simulink model "eVTOL_System"  (R2024b)
settings: Solver=FixedStepAuto  StartTime=0.0  StopTime=inf  RelTol=1e-3
undefined symbols (not defined in the file): airspeed, Battery, BCE12, BCE_Set_init, BMS_Controller_State, C, Cell10_P, Cell11_P, Cell12_P, Cell13_P, Cell14_P, Cell15_P, Cell16_P, Cell17_P, Cell18_P, Cell19_P, Cell1_N, Cell1_P, Cell20_P, Cell21_P, Cell22_P, Cell23_P, Cell24_P, Cell2_P, Cell3_P, Cell4_P, Cell5_P, Cell6_P, Cell7_P, Cell8_P, Cell9_P, Charging_State, CityMission, control, controlParams, ControlSampleTime, CriticalTiltAngle, currentFactor, CV_Gain, ddx, ddy, ddz, Device_01, Device_02, DiscIntNeverNeededParam, dx, dy, dz, Earth, env, F, F28379D_ADC_MaxCount, F28379D_ADC_Vmax, FixedWingMission, flightState, Foc_Ki_IxTcpu, Foc_Ki_S, Foc_Kp_I, Foc_Kp_S, fractalcoef ... (+68)
libraries: fl_lib x1115, nesl_utility x617, slrealtimeethercatlib x217, simulink x130, canmsglib x101, speedgoatlib_IO611_obsolete x91, slpidlib x49, mcbcontrolslib x44, slrealtimeutilitieslib x35, speedgoatlib_hdlCoder_IO3xx x31, dspstat3 x24, mcbpositiondecoderlib x12
(part 4 of 31)

== system eVTOL_System/User Interface/Motor Drive User Interface ==
  note: Fault Present
  note: Hardware-in-the-Loop
      | Motor & Inverter
      | Real-Time Simulation
  note: Motor Currents [A]
  note: Model Response
  note: Kp
  note: UI Speed Command enabled
  note: Tx: Message to Controller
  note: Speed Controller PI Gain Tuning
  note: Ki
  note: Rx: Message From Controller
  note: Open A-
  note: Open C-
  note: Short AB
  note: Short B
  note: Short CA
  note: Open A+
  note: Short BC
  note: Open B-
  note: Open B+
  note: Open C+
  note: Short A
  note: Short C
  note: Inverter Faults
  note: Motor Speed [rpm]
  note: Time [s]
  note: Time [s]
  note: Time [s]
  note: Motor Speed [rpm]
  note: Encoder Count [steps]
  note: (only for switching inverter)
  note: (only short A with included bitstream)
  note: Motor Drive User Interface
  Dashboard Scope1 : DashboardScope  ShowInitialText=off  TimeSpan=0.10000000000000001  Ymin=-50  Ymax=50  ScaleAtStop=off  UpdateMode=Scroll
  Dashboard Scope2 : DashboardScope  ShowInitialText=off  TimeSpan=1  Ymin=0  Ymax=1e5  ScaleAtStop=off
  Dashboard Scope3 : DashboardScope  ShowInitialText=off  TimeSpan=10  Ymin=0  Ymax=3000  ScaleAtStop=off
  Edit : EditField  LabelPosition=Hide  ShowInitialText=on  Alignment=Center
  Edit1 : EditField  LabelPosition=Hide  ShowInitialText=on  Alignment=Center
  Faults Enabled : SliderSwitchBlock  LabelPosition=Hide
      settings: Values={{'Faults UI OFF', 'Faults UI ON'}, [0 1]}
  Gauge1 : CircularGaugeBlock  LabelPosition=Hide  ScaleMin=-1500  ScaleMax=1500
  Lamp2 : LampBlock  LabelPosition=Hide
  Lamp3 : LampBlock  LabelPosition=Hide
  Lamp4 : LampBlock  LabelPosition=Hide
  Open An : ToggleSwitchBlock  LabelPosition=Hide
      settings: Values={{'Off', 'On'}, [0 1]}
  Open Ap : ToggleSwitchBlock  LabelPosition=Hide
      settings: Values={{'Off', 'On'}, [0 1]}
  Open Bn : ToggleSwitchBlock  LabelPosition=Hide
      settings: Values={{'Off', 'On'}, [0 1]}
  Open Bp : ToggleSwitchBlock  LabelPosition=Hide
      settings: Values={{'Off', 'On'}, [0 1]}
  Open Cn : ToggleSwitchBlock  LabelPosition=Hide
      settings: Values={{'Off', 'On'}, [0 1]}
  Open Cp : ToggleSwitchBlock  LabelPosition=Hide
      settings: Values={{'Off', 'On'}, [0 1]}
  Short A : ToggleSwitchBlock  LabelPosition=Hide
      settings: Values={{'Off', 'On'}, [0 1]}
  Short AB : ToggleSwitchBlock  LabelPosition=Hide
      settings: Values={{'Off', 'On'}, [0 1]}
  Short B : ToggleSwitchBlock  LabelPosition=Hide
      settings: Values={{'Off', 'On'}, [0 1]}
  Short BC : ToggleSwitchBlock  LabelPosition=Hide
      settings: Values={{'Off', 'On'}, [0 1]}
  Short C : ToggleSwitchBlock  LabelPosition=Hide
      settings: Values={{'Off', 'On'}, [0 1]}
  Short CA : ToggleSwitchBlock  LabelPosition=Hide
      settings: Values={{'Off', 'On'}, [0 1]}
  Slider : SliderBlock  LabelPosition=Hide  ScaleMin=1e-5  ScaleMax=10  ScaleType=Log
  Slider Switch : SliderSwitchBlock  LabelPosition=Hide
      settings: Values={{'Sinus Open Loop', 'FOC Closed Loop'}, [0 1]}
  Slider Switch1 : SliderSwitchBlock  LabelPosition=Hide
      settings: Values={{'PWM OFF', 'PWM ON'}, [0 1]}
  Slider Switch2 : SliderSwitchBlock  LabelPosition=Hide
      settings: Values={{'Default Values', 'Live Tuning'}, [1 0]}
  Slider1 : SliderBlock  LabelPosition=Hide  ScaleMin=1e-5  ScaleMax=10  ScaleType=Log

== system eVTOL_System/Visualization/No Visualization ==
  UAVState : Inport
  Terminator : Terminator
  wires:
  UAVState/1 -> Terminator/1

== system eVTOL_System/Visualization/Photorealistic ==
  UAVState : Inport
  PhotorealisticHIL : Subsystem  VariantControl=Visualization==2 && str2num(get_param(['eVTOL_System/Motor Drive/SimulationVariant'], 'Value'))~=1
  PhotorealisticMIL : Subsystem  VariantControl=Visualization==2 && str2num(get_param(['eVTOL_System/Motor Drive/SimulationVariant'], 'Value'))==1

== system eVTOL_System/Visualization/Visualization ==
  UAVState : Inport
  VisualizationHIL : Subsystem  VariantControl=Visualization==1 && (str2num(get_param(['eVTOL_System/Motor Drive/SimulationVariant'], 'Value'))~=1)
  VisualizationMIL : Subsystem  VariantControl=Visualization == 1 && (str2num(get_param(['eVTOL_System/Motor Drive/SimulationVariant'], 'Value'))==1)

== system eVTOL_System/Battery System/BMS/HIL ==
  State_Request : Inport  OutDataTypeStr=Enum: SRE  PortDimensions=1
  Sensor_Values : Inport  Port=2
  Bus Creator : BusCreator  Inputs=4  OutDataTypeStr=Bus: Controller_Info  NonVirtualBus=on
      settings: InheritFromInputs=off
  Bus Creator1 : BusCreator  Inputs=3  OutDataTypeStr=Bus: Controller_Output  NonVirtualBus=on
      settings: InheritFromInputs=off
  Cell Monitoring Unit : Subsystem
  Controller_100Cells : Subsystem  VariantControl=Ns_Module == 12
  Controller_76Cells : Subsystem  Commented=on
  Rate Transition : RateTransition  OutPortSampleTime=ts_controller
  Rate Transition1 : RateTransition  InitialCondition=SRE.Standby  OutPortSampleTime=ts_controller
  Rate Transition3 : RateTransition  Commented=on  InitialCondition=SRE.Standby  OutPortSampleTime=ts_controller
  Simscape Bus : SimscapeBus
  Terminator{,1..6} (7 alike) : Terminator
  Cells : PMIOPort  Side=Left
  Cells1 : PMIOPort  Port=2  Side=Left
  Cells2 : PMIOPort  Port=3  Side=Left
  Controller_Info : Outport
  Controller_Output : Outport  Port=2  OutDataTypeStr=Bus: Controller_Output  VectorParamsAs1DForOutWhenUnconnected=off  BusOutputAsStruct=on
  wires:
  Bus Creator/1 -> Controller_Info/1  "Controller_Info"
  Bus Creator1/1 -> Controller_Output/1  "Controller_Output"
  Rate Transition/1 -> Cell Monitoring Unit/2(Sensor_Values)
  Cell Monitoring Unit/1(Sensor Values) -> Controller_100Cells/1(Sensor_Values)
  Rate Transition1/1 -> Controller_100Cells/2(State_Request)
  Controller_100Cells/1(BMS_Faults) -> Bus Creator/1
  Controller_100Cells/2(Charging_State) -> Bus Creator/2
  Controller_100Cells/3(BMS_State) -> Bus Creator/3
  Controller_100Cells/4(SOC) -> Bus Creator/4
  Controller_100Cells/5(Discharge_Current_Limit) -> Bus Creator1/1
  Controller_100Cells/6(Charge_Current_Limit) -> Bus Creator1/2
  Controller_100Cells/7(Charge_Current_Req) -> Bus Creator1/3
  State_Request/1 -> Rate Transition1/1
  Sensor_Values/1 -> Rate Transition/1
  Rate Transition3/1 -> Controller_76Cells/2(State_Request)
  Controller_76Cells/1(Faults) -> Terminator/1
  Controller_76Cells/2(Charging_State) -> Terminator1/1  "Charging_State"
  Controller_76Cells/3(BMS_Controller_State) -> Terminator2/1  "BMS_State"
  Controller_76Cells/4(SOC) -> Terminator3/1
  Controller_76Cells/5(Discharge_Current_Limit) -> Terminator4/1
  Controller_76Cells/6(Charge_Current_Limit) -> Terminator5/1
  Controller_76Cells/7(Charge_Current_Req) -> Terminator6/1
  [Bal_Cmd_Controller1] -> Cell Monitoring Unit/1(Bal_Cmd_Controller)
  Controller_100Cells/8(Bal_Cmd_76Cells) -> [Bal_Cmd_Controller1]
  connections:
  Simscape Bus/RConn1 -- Cells/RConn1
  Cells1/RConn1 -- Cell Monitoring Unit/LConn1
  Cells2/RConn1 -- Cell Monitoring Unit/LConn2

== system eVTOL_System/Battery System/BMS/MIL ==
  State_Request : Inport  OutDataTypeStr=Enum: SRE  PortDimensions=1
  Sensor_Values : Inport  Port=2  OutDataTypeStr=Bus: Sensor_Values  BusOutputAsStruct=on
  Bus Creator : BusCreator  Inputs=4  OutDataTypeStr=Bus: Controller_Info  NonVirtualBus=on
      settings: InheritFromInputs=off
  Bus Creator1 : BusCreator  Inputs=4  OutDataTypeStr=Bus: Controller_Output  NonVirtualBus=on
      settings: InheritFromInputs=off
  Cell Monitoring Unit : Subsystem
  Controller : Subsystem
  Rate Transition : RateTransition  InitialCondition=struct('Cell_Voltages',3.7*ones(Ns_Module,1),'Cell_Temperatures',298.15*ones(Ns_Module,1),'Pack_Current',0,'Pack_Voltage',3.7*Ns_Module)  OutPortSampleTime=ts_controller
  Rate Transition1 : RateTransition  InitialCondition=SRE.Standby  OutPortSampleTime=ts_controller
  Rate Transition2 : RateTransition  Commented=on  InitialCondition=struct('Cell_Voltages',3.7*ones(1,Ns_Module),'Cell_Temperatures',298.15*ones(1,Ns_Module),'Pack_Current',0,'Pack_Voltage',3.7*Ns_Module)  OutPortSampleTime=ts_controller
  Rate Transition3 : RateTransition  OutPortSampleTime=ts_system
  Rate Transition{4..7} (4 alike) : RateTransition
  Cells : PMIOPort  Side=Left
  Cells1 : PMIOPort  Port=2  Side=Left
  Cells2 : PMIOPort  Port=3  Side=Left
  Controller_Info : Outport
  Controller_Output : Outport  Port=2  OutDataTypeStr=Bus: Controller_Output  VectorParamsAs1DForOutWhenUnconnected=off  BusOutputAsStruct=on
  wires:
  Bus Creator/1 -> Controller_Info/1  "Controller_Info"
  Bus Creator1/1 -> Rate Transition3/1  "Controller_Output"
  State_Request/1 -> Rate Transition1/1
  Controller/1(Faults) -> Bus Creator/1
  Controller/2(Charging_State) -> Bus Creator/2  "Charging_State"
  Controller/3(BMS_Controller_State) -> Bus Creator/3  "BMS_State"
  Controller/4(SOC) -> Bus Creator/4
  Controller/5(Discharge_Current_Limit) -> Rate Transition7/1
  Controller/6(Charge_Current_Limit) -> Rate Transition5/1
  Controller/7(Charge_Current_Req) -> Rate Transition4/1
  Controller/8(Bal_Cmd) -> Rate Transition6/1, [Bal_Cmd_Controller]
  [Bal_Cmd_Controller] -> Cell Monitoring Unit/1(Bal_Cmd_Controller)
  Sensor_Values/1 -> Rate Transition/1
  Cell Monitoring Unit/1(Sensor Values) -> Controller/1(Sensor_Values)
  Rate Transition1/1 -> Controller/2(State_Request)
  Rate Transition/1 -> Cell Monitoring Unit/2(Sensor_Values)
  Rate Transition3/1 -> Controller_Output/1
  Rate Transition4/1 -> Bus Creator1/3
  Rate Transition6/1 -> Bus Creator1/4
  Rate Transition5/1 -> Bus Creator1/2
  Rate Transition7/1 -> Bus Creator1/1
  connections:
  Cells/RConn1 -- Cell Monitoring Unit/LConn1
  Cells1/RConn1 -- Cell Monitoring Unit/LConn2
  Cells2/RConn1 -- Cell Monitoring Unit/LConn3

== system eVTOL_System/Battery System/Battery/Battery Pack ==
  Ambient_Temperature : Inport
  100-Cell : Subsystem  VariantControl=Ns_Module == 12
  Batt+ : PMIOPort  Side=Right
  Batt- : PMIOPort  Port=2  Side=Right
  Cells : PMIOPort  Port=3  Side=Right
  Cells1 : PMIOPort  Port=4  Side=Right
  Cells2 : PMIOPort  Port=5  Side=Right
  Cell_Voltages : Outport
  Cell_Temperatures : Outport  Port=2
  Cell_SOCs : Outport  Port=3
  wires:
  Ambient_Temperature/1 -> 100-Cell/1(Ambient_Temperature)
  100-Cell/1(Cell_Voltages) -> Cell_Voltages/1
  100-Cell/2(Cell_Temperatures) -> Cell_Temperatures/1
  100-Cell/3(Cell_SOCs) -> Cell_SOCs/1
  connections:
  100-Cell/RConn1 -- Batt+/RConn1
  100-Cell/RConn2 -- Batt-/RConn1
  100-Cell/RConn3 -- Cells/RConn1
  Cells1/RConn1 -- 100-Cell/RConn4
  Cells2/RConn1 -- 100-Cell/RConn5

== system eVTOL_System/Battery System/Battery/Electrical Interface ==
  Current_Request : Inport
  Controlled Current Source : fl_lib/Electrical/Electrical Sources/Controlled Current Source
  Current Sensor : fl_lib/Electrical/Electrical Sensors/Current Sensor
  Data Type Conversion : DataTypeConversion  OutDataTypeStr=double  SaturateOnIntegerOverflow=off  RndMeth=Floor
  Electrical Reference : fl_lib/Electrical/Electrical Elements/Electrical Reference
  PS-Simulink Converter : nesl_utility/PS-Simulink Converter  PhysicalDomain=network_engine_domain  SubClassName=ps_output  LeftPortType=input  RightPortType=output  PseudoPeriodic=off  Frequencies=[]  VectorFormat=inherit  Unit=inherit  AffineConversion=off
  PS-Simulink Converter1 : nesl_utility/PS-Simulink Converter  PhysicalDomain=network_engine_domain  SubClassName=ps_output  LeftPortType=input  RightPortType=output  PseudoPeriodic=off  Frequencies=[]  VectorFormat=inherit  Unit=inherit  AffineConversion=off
  Simulink-PS Converter3 : nesl_utility/Simulink-PS Converter  PhysicalDomain=network_engine_domain  SubClassName=ps_input  LeftPortType=input  RightPortType=output  PseudoPeriodic=off  Frequencies=[]  NoiseDistribution=none  NoiseParameters=[]  Unit=1  AffineConversion=off  FilteringAndDerivatives=zero  SimscapeFilterOrder=1  InputFilterTimeConstant=0.001  UdotUserProvided=1
  Solver Configuration : nesl_utility/Solver Configuration  PhysicalDomain=network_engine_domain  SubClassName=solver  LeftPortType=input  RightPortType=generic  Tones=[]  Harmonics=[]  SimulateNoise=off  Profile=off  UseLocalSampling=off  EnableSwitchedLinearOptims=on  FrequencyDomain=off  UseCCode=off  RelTol=0.001  AbsTol=0.001  MinStep=1e-09  ToWorkspace=off  RevertToSquareIcSolve=off  NumHomotopyIterations=100  PhasorMode=off  PhasorModeNumHarmonics=1  ConsistencySolver=NEWTON_XTOL_AFTER_FTOL  IndexReductionMethod=DerivativeReplacement  DoDC=off  ResidualTolerance=1e-09  ConsistencyTolSource=GLOBAL  ConsistencyAbsTol=0.001  ConsistencyRelTol=0.001  ConsistencyTolFactor=1e-09  UseLocalSolver=on  LocalSolverChoice=NE_BACKWARD_EULER_ADVANCER  ResolveIndetEquations=on  FunctionEvalNumThread=1  LocalSolverSampleTime=ts_system  DoFixedCost=on  MaxNonlinIter=3  MaxModeIter=2  ComputeImpulses=off  ImpulseIterations=2  LinearAlgebra=auto  LinearAlgebraNumThread=0  EquationFormulation=NE_TIME_EF  DelaysMemoryBudget=1024  AutomaticFiltering=on  FilteringTimeConstant=0.001  PartitionStorageMethod=AS_NEEDED  PartitionMemoryBudget=1024  PartitionMethod=ROBUST  MultibodyUseLocalSolver=off  MultibodyLocalSolverChoice=ODE1  MultibodyLocalSolverSampleTime=0.001
  Voltage Sensor7 : fl_lib/Electrical/Electrical Sensors/Voltage Sensor
      settings: LibrarySourceBlock=BatteryPack_lib/CellMonitoringUnit/Voltage Sensor1
  Batt+ : PMIOPort  Side=Left
  Batt- : PMIOPort  Port=2  Side=Left
  Pack_Current : Outport
  Pack_Voltage : Outport  Port=2
  wires:
  Current_Request/1 -> Data Type Conversion/1
  PS-Simulink Converter1/1 -> Pack_Current/1
  PS-Simulink Converter/1 -> Pack_Voltage/1
  Data Type Conversion/1 -> Simulink-PS Converter3/1
  connections:
  Controlled Current Source/LConn1 -- Voltage Sensor7/LConn1 -- Batt+/RConn1
  Current Sensor/RConn2 -- Solver Configuration/RConn1 -- Electrical Reference/LConn1 -- Controlled Current Source/RConn2
  PS-Simulink Converter1/LConn1 -- Current Sensor/RConn1
  Simulink-PS Converter3/RConn1 -- Controlled Current Source/RConn1
  Batt-/RConn1 -- Voltage Sensor7/RConn2 -- Current Sensor/LConn1
  Voltage Sensor7/RConn1 -- PS-Simulink Converter/LConn1

== system eVTOL_System/Battery System/Battery/HW Interface ==
  Sensor_Values_Sim : Inport
  BCE - HIL : Subsystem  VariantControl=strcmp(get_param(['eVTOL_System/Battery System/Instrumentation/Simulation_Profile_Value'], 'Value'),'1')
  MIL : Subsystem  VariantControl=strcmp(get_param(['eVTOL_System/Battery System/Instrumentation/Simulation_Profile_Value'], 'Value'),'0')
  Cells_IN : PMIOPort  Side=Left
  Cells_OUT : PMIOPort  Port=2  Side=Right
  Sensor_Values_Real : Outport

== system eVTOL_System/Battery System/Battery/Override ==
  Input : Inport
  BrokenWireReset : Constant  Value=0  OutDataTypeStr=boolean  SampleTime=-1
  Broken_Wire_Fault : Constant  Value=0  SampleTime=-1
  Bus Creator : BusCreator  Inputs=6  OutDataTypeStr=Bus: Sensor_Values
  Cell Number : Constant  Value=12  SampleTime=-1
  Celsius_to_Kelvin : Subsystem
  Delay{,1..3} (4 alike) : Delay  DelayLength=1
  MATLAB Function : MATLAB Function  TreatAsAtomicUnit=on
  Rate Transition : RateTransition
  Reset : Constant  Value=0  SampleTime=-1
  TEnable : Constant  OutDataTypeStr=boolean  SampleTime=-1
  TValue : Constant  Value=25  SampleTime=-1
  UpdateTempValue : Constant  Value=NaN  SampleTime=-1
  UpdateVoltageValue : Constant  Value=NaN
  VEnable : Constant  OutDataTypeStr=boolean  SampleTime=-1
  VValue : Constant  Value=2.5  SampleTime=-1
  Output : Outport
  wires:
  TEnable/1 -> MATLAB Function/6(TEnable)
  MATLAB Function/7(TArrayFb) -> Delay1/1
  Input/1 -> Rate Transition/1
  VEnable/1 -> MATLAB Function/5(VEnable)
  UpdateVoltageValue/1 -> MATLAB Function/7(UpdateVValue)
  Reset/1 -> MATLAB Function/10(Reset)
  MATLAB Function/1(Output1) -> Bus Creator/1  "Cell_Voltages"
  MATLAB Function/8(VArrayFb) -> Delay/1
  Delay1/1 -> MATLAB Function/12(TArray)
  MATLAB Function/2(Output2) -> Bus Creator/2  "Cell_Temperatures"
  MATLAB Function/3(Output3) -> Bus Creator/3  "Pack_Current"
  MATLAB Function/4(Output4) -> Bus Creator/4  "Pack_Voltage"
  MATLAB Function/5(Output5) -> Bus Creator/5  "Pack_Voltage1"
  MATLAB Function/6(Output6) -> Bus Creator/6  "Pack_Voltage2"
  Bus Creator/1 -> Output/1
  Delay/1 -> MATLAB Function/13(VArray)
  VValue/1 -> MATLAB Function/2(VValue)
  Cell Number/1 -> MATLAB Function/1(CellNumber)
  TValue/1 -> Celsius_to_Kelvin/1(C)
  UpdateTempValue/1 -> MATLAB Function/8(UpdateTValue)
  Celsius_to_Kelvin/1(K) -> MATLAB Function/3(TValue)
  Broken_Wire_Fault/1 -> MATLAB Function/9(Broken_wire)
  BrokenWireReset/1 -> MATLAB Function/11(Wire_reset)
  MATLAB Function/9(flagFb) -> Delay2/1
  MATLAB Function/10(BrokenWireFb) -> Delay3/1
  Delay2/1 -> MATLAB Function/14(flag)
  Delay3/1 -> MATLAB Function/15(BrokenWires)
  Rate Transition/1 -> MATLAB Function/4(InputVal)

== system eVTOL_System/Battery System/Instrumentation/Celsius_to_Kelvin ==
  C : Inport
  Add : Sum
  Constant4 : Constant  Value=273.15
  K : Outport
  wires:
  Constant4/1 -> Add/2
  C/1 -> Add/1
  Add/1 -> K/1

== system eVTOL_System/Battery System/Instrumentation/Current Control ==
  Current_Request_User : Inport
  Current_Request_User_Bypass : Inport  Port=2
  Controller_Info : Inport  Port=3
  Controller_Output : Inport  Port=4
  Bus Selector : BusSelector  OutputSignals=Charge_Current_Limit,Discharge_Current_Limit
  Bus Selector1 : BusSelector  OutputSignals=BMS_State
  Compare To Constant : simulink/Logic and Bit Operations/Compare To Constant  relop===  const=BMS_Controller_State.BMS_Fault  OutDataTypeStr=uint8
  Current_Req : Constant  Value=0  SampleTime=ts_controller
  Saturation Dynamic : simulink/Discontinuities/Saturation Dynamic  OutMin=[]  OutMax=[]  OutDataTypeStr=Inherit: Same as second input  OutDataType=fixdt(1, 16)  OutScaling=2^-10  DoSatur=off
  Switch : Switch  Criteria=u2 > Threshold  SaturateOnIntegerOverflow=off  InputSameDT=off
  Switch1 : Switch  Criteria=u2 > Threshold  SaturateOnIntegerOverflow=off  InputSameDT=off
  Current_Request : Outport
  wires:
  Current_Request_User/1 -> Saturation Dynamic/2, Switch1/1
  Controller_Output/1 -> Bus Selector/1
  Bus Selector/1 -> Saturation Dynamic/1  "<Charge_Current_Limit>"
  Bus Selector/2 -> Saturation Dynamic/3  "<Discharge_Current_Limit>"
  Current_Req/1 -> Switch/1
  Saturation Dynamic/1 -> Switch/3
  Controller_Info/1 -> Bus Selector1/1
  Bus Selector1/1 -> Compare To Constant/1  "<BMS_State>"
  Switch1/1 -> Current_Request/1
  Switch/1 -> Switch1/3
  Current_Request_User_Bypass/1 -> Switch1/2
  Compare To Constant/1 -> Switch/2

== system eVTOL_System/Battery System/Instrumentation/Instrumented Signals ==
  Controller_Output : Inport
  Controller_Info : Inport  Port=2
  Sensor_Values : Inport  Port=3
  Balancing_Currents : Inport  Port=4
  Cells_SOCs : Inport  Port=5
  100-Cell : Subsystem  VariantControl=Ns_Module == 12
  wires:
  Controller_Output/1 -> 100-Cell/1(Controller_Output)
  Controller_Info/1 -> 100-Cell/2(Controller_Info)
  Sensor_Values/1 -> 100-Cell/3(Sensor_Values)
  Balancing_Currents/1 -> 100-Cell/4(Balancing_Currents)
  Cells_SOCs/1 -> 100-Cell/5(Cells_SOCs)

== system eVTOL_System/Dynamics/Force and Moments/Aerodynamic Drag ==
  DCM_be : Inport
  Vb : Inport  Port=2
  Constant : Constant  Value=windVel
  Constant1 : Constant  Value=uavParam.aero.dragCoeffMov
  calcDragVector : MATLAB Function  TreatAsAtomicUnit=on
  gain : Gain  Gain=-1
  relative air velocity (body frame) : Sum
  wind (body frame) : Product  Multiplication=Matrix(*)
  F_d : Outport
  wires:
  Vb/1 -> gain/1
  calcDragVector/1(dragVec) -> F_d/1
  relative air velocity (body frame)/1 -> calcDragVector/1(airVel)
  gain/1 -> relative air velocity (body frame)/2
  Constant1/1 -> calcDragVector/2(dragCoeff)
  DCM_be/1 -> wind (body frame)/1
  Constant/1 -> wind (body frame)/2
  wind (body frame)/1 -> relative air velocity (body frame)/1

== system eVTOL_System/Dynamics/Force and Moments/Aerodynamic Forces ==
  Wind_e : Inport
  Rho : Inport  Port=2
  CtrlSurfaces : Inport  Port=3
  UAVState : Inport  Port=4
  Bus Selector2 : BusSelector  OutputSignals=Ve,Euler,pqr
  Compute Air Data : Subsystem  TreatAsAtomicUnit=on  VariantControl=use_aerospace_blocks == 1
  Compute Body Frame Forces and Moments : Subsystem
  Rotate Vw : Subsystem
  Vair : Sum  Inputs=-+  InputSameDT=on  SaturateOnIntegerOverflow=on  OutDataTypeStr=Inherit: Same as first input
  AirData : Outport  VectorParamsAs1DForOutWhenUnconnected=off
  F : Outport  Port=2
  M : Outport  Port=3
  wires:
  Bus Selector2/1 -> Vair/2  "<Ve>"
  UAVState/1 -> Bus Selector2/1
  Compute Body Frame Forces and Moments/1(F_b) -> F/1
  Wind_e/1 -> Vair/1
  CtrlSurfaces/1 -> Compute Body Frame Forces and Moments/2(CtrlSurfaces)
  Compute Air Data/1(AirData) -> AirData/1, Compute Body Frame Forces and Moments/1(AirData)
  Bus Selector2/3 -> Compute Body Frame Forces and Moments/3(p,q,r)  "<pqr>"
  Compute Body Frame Forces and Moments/2(M_b) -> M/1
  Rotate Vw/1(Vb) -> Compute Air Data/1(Vb)
  Rho/1 -> Compute Air Data/2(Rho)
  Bus Selector2/2 -> Rotate Vw/2(Euler)  "<Euler>"
  Vair/1 -> Rotate Vw/1(Vw)

== system eVTOL_System/Dynamics/Force and Moments/Gravity ==
  DCM_be : Inport
  Constant : Constant  Value=[0 0 uavParam.aero.g]'
  Gain : Gain  Gain=uavParam.geom.mass
  Matrix Multiply : Product  Multiplication=Matrix(*)
  F_g : Outport
  wires:
  Matrix Multiply/1 -> Gain/1
  Constant/1 -> Matrix Multiply/2
  DCM_be/1 -> Matrix Multiply/1
  Gain/1 -> F_g/1

== system eVTOL_System/Dynamics/Force and Moments/Propulsion ==
  note: TurnDirection : Propeller spin direction, specified as 3 element vector of the form [x y z] where each element are axis directions in the x,y,z direction of the rotor coordinate (front - right - down)
      |
      | Example: [0 0 -1] would set the propeller to spin around the positive z direction (Counter-clockwise when seen from above)
  note: RotorDirection : Rotor tilt direction, specified as 3 element vector of the form [x y z] where each element are directions in the x,y,z direction of the body coordinate (front - right - down)
      |
      | example : [0 0 -1] would set the rotor in the negative z direction (vertical upwards)
  note: Rotor Numbering :
      | Rotor 1 : Front left
      | Rotor 2 : Front right
      | Rotor 3 : Rear right
      | Rotor 4 : Rear left
  note: Tilt Rotors Dynamics
  note: Sum of Moments
  note: Rotor 1
      | (tiltrotor)
  note: Rotors
  note: Rotor 2
      | (titlrotor)
  note: Rotor 3
  note: Rotor 4
  note: Sum of Forces
  note: Rotor Parameters
  Bus Element In : Inport  PortName=Actuator  Element=w1
  Bus Element In1 : Inport  PortName=Actuator  Element=Tilt1
  Bus Element In2 : Inport  PortName=Actuator  Element=Tilt2
  Bus Element In3 : Inport  PortName=Actuator  Element=w2
  Bus Element In5 : Inport  PortName=Actuator  Element=w4
  Bus Element In4 : Inport  PortName=Actuator  Element=w3
  In Bus Element{,2,4,6} (4 alike) : Inport  Port=2  PortName=States  Element=Vb
  In Bus Element{1,3,5,7} (4 alike) : Inport  Port=2  PortName=States  Element=pqr
  Add : Sum  Inputs=++++
  Add1 : Sum  Inputs=++++
  Bus Creator : BusCreator  Inputs=6
  Constant : Constant  Value=uavParam.geom.RotorArm1
  Constant1 : Constant  Value=0
  Constant10 : Constant  Value=uavParam.geom.RotorArm4
  Constant11 : Constant  Value=[0 0 -1]
  Constant13 : Constant  Value=[ 0; 0; 1]
  Constant2 : Constant  Value=0
  Constant3 : Constant  Value=uavParam.geom.RotorArm2
  Constant5 : Constant  Value=[ 0; 0; 1]
  Constant6 : Constant  Value=uavParam.geom.RotorArm3
  Constant7 : Constant  Value=[0 0 -1]
  Constant8 : Constant  Value=[ 0; 0; -1]
  Constant9 : Constant  Value=[ 0; 0; -1]
  Cos1 : Trigonometry  Operator=cos
  Cos2 : Trigonometry  Operator=cos
  Gain : Gain  Gain=-1
  Gain1 : Gain  Gain=-1
  Model{,1..3} (4 alike) : ModelReference  ModelNameDialog=PropellerDynamics.slx  SimulationMode=Normal  ModelReferenceVersion=4.5
  Mux : Mux  Inputs=3
  Mux1 : Mux  Inputs=3
  Rate Transition : RateTransition
  Rate Transition1 : RateTransition
  Sin1 : Trigonometry
  Sin2 : Trigonometry
  Tilt Servo Dynamics : Subsystem
  Transfer Fcn{,1..3} (4 alike) : TransferFcn  Denominator=[0.1 1]
  RotorParameters : Outport
  M : Outport  Port=2
  F : Outport  Port=3
  wires:
  In Bus Element/1 -> Model/2
  In Bus Element1/1 -> Model/3
  Constant/1 -> Model/4
  Sin2/1 -> Mux/1
  Cos1/1 -> Gain/1
  Constant1/1 -> Mux/2
  Gain/1 -> Mux/3
  Mux/1 -> Rate Transition/1
  Cos2/1 -> Gain1/1
  Sin1/1 -> Mux1/1
  Constant2/1 -> Mux1/2
  Mux1/1 -> Rate Transition1/1
  [TiltArm1] -> Model/5
  Add/1 -> F/1
  Gain1/1 -> Mux1/3
  Constant8/1 -> Model/6
  Model/1 -> [F1]
  Model/2 -> [M1]
  Model1/1 -> [F2]
  In Bus Element2/1 -> Model1/2
  Constant3/1 -> Model1/4
  Constant5/1 -> Model1/6
  [TiltArm2] -> Model1/5
  In Bus Element3/1 -> Model1/3
  Model1/2 -> [M2]
  Model2/1 -> [F3]
  In Bus Element4/1 -> Model2/2
  Constant6/1 -> Model2/4
  Constant9/1 -> Model2/6
  Constant7/1 -> Model2/5
  In Bus Element5/1 -> Model2/3
  Model2/2 -> [M3]
  Model3/1 -> [F4]
  In Bus Element6/1 -> Model3/2
  Constant10/1 -> Model3/4
  Constant13/1 -> Model3/6
  Constant11/1 -> Model3/5
  In Bus Element7/1 -> Model3/3
  Model3/2 -> [M4]
  [F1] -> Add/1
  [F2] -> Add/2
  [F3] -> Add/3
  [F4] -> Add/4
  [M4] -> Add1/4
  Add1/1 -> M/1
  [M3] -> Add1/3
  [M2] -> Add1/2
  [M1] -> Add1/1
  Model/3 -> Transfer Fcn/1
  Model1/3 -> Transfer Fcn1/1
  Model2/3 -> Transfer Fcn2/1
  Model3/3 -> Transfer Fcn3/1
  [w1] -> Bus Creator/1  "w1"
  [w2] -> Bus Creator/2  "w2"
  [w3] -> Bus Creator/3  "w3"
  [w4] -> Bus Creator/4  "w4"
  Bus Creator/1 -> RotorParameters/1
  [RotorA] -> Bus Creator/5  "Rotor A"
  [RotorB] -> Bus Creator/6  "Rotor B"
  Bus Element In/1 -> Model/1
  Bus Element In3/1 -> Model1/1
  Bus Element In4/1 -> Model2/1
  Bus Element In5/1 -> Model3/1
  Tilt Servo Dynamics/1(Tilt1) -> Cos1/1, Sin2/1, [RotorA]
  Tilt Servo Dynamics/2(Tilt2) -> Sin1/1, Cos2/1, [RotorB]
  Bus Element In1/1 -> Tilt Servo Dynamics/1(TiltA)
  Bus Element In2/1 -> Tilt Servo Dynamics/2(TiltB)
  Transfer Fcn/1 -> [w1]
  Transfer Fcn1/1 -> [w2]
  Transfer Fcn2/1 -> [w3]
  Transfer Fcn3/1 -> [w4]
  Rate Transition/1 -> [TiltArm1]
  Rate Transition1/1 -> [TiltArm2]

== system eVTOL_System/Dynamics/Force and Moments/Weather Model ==
  AirData : Inport
  Xe : Inport  Port=2
  Euler : Inport  Port=3
  Simple Model : Subsystem  VariantControl=Wind==0
  Weather Model : Subsystem  VariantControl=Wind==1
  Wind_e : Outport
  Rho : Outport  Port=2

== system eVTOL_System/Dynamics/Variant Subsystem/No Sensors ==
  Bus Element In9 : Inport  PortName=UAVStates  Element=Ve
  Bus Element In11 : Inport  PortName=UAVStates  Element=Ve
  Bus Element In2 : Inport  PortName=UAVStates  Element=Xe
  Bus Element In3 : Inport  PortName=UAVStates  Element=Euler
  Bus Element In8 : Inport  PortName=UAVStates  Element=Euler
  Bus Element In4 : Inport  PortName=UAVStates  Element=DCMbe
  Bus Element In5 : Inport  PortName=UAVStates  Element=pqr
  Bus Element In6 : Inport  PortName=UAVStates  Element=Vb
  Bus Element In7 : Inport  PortName=UAVStates  Element=Abb
  Bus Element In10 : Inport  PortName=UAVStates  Element=RotorParameters
  Bus Element In : Inport  PortName=UAVStates  Element=airspeed
  Bus Element In12 : Inport  PortName=UAVStates  Element=gndspeed
  Bus Element In1 : Inport  PortName=UAVStates  Element=course
  Bus Creator : BusCreator  Inputs=14
  Direction Cosine Matrix to Quaternions1 : sharedtransform/Direction Cosine Matrix  to Quaternions  aMode=0  action=None  tolerance=eps(2)
      settings: LibrarySourceBlock=|
      | aerolibtransform2/Direction Cosine Matrix
      | to Quaternions
  MATLAB Function : MATLAB Function  TreatAsAtomicUnit=on
  SensorData : Outport
  wires:
  Bus Element In8/1 -> MATLAB Function/1(euler)  "Euler"
  Bus Creator/1 -> SensorData/1
  Bus Element In5/1 -> Bus Creator/8  "pqr"
  Bus Element In2/1 -> Bus Creator/4  "Xe"
  MATLAB Function/1(ypr) -> Bus Creator/13
  Bus Element In9/1 -> Bus Creator/5  "Ve"
  Bus Element In/1 -> Bus Creator/3  "airspeed"
  Bus Element In4/1 -> Bus Creator/6, Direction Cosine Matrix to Quaternions1/1  "DCMbe"
  Direction Cosine Matrix to Quaternions1/1 -> Bus Creator/7
  Bus Element In6/1 -> Bus Creator/9  "Vb"
  Bus Element In7/1 -> Bus Creator/10  "Abb"
  Bus Element In10/1 -> Bus Creator/12  "RotorParameters"
  Bus Element In3/1 -> Bus Creator/11  "Euler"
  Bus Element In11/1 -> Bus Creator/14  "Ve_ground"
  Bus Element In12/1 -> Bus Creator/2  "gndspeed"
  Bus Element In1/1 -> Bus Creator/1  "course"

== system eVTOL_System/Dynamics/Variant Subsystem/Sensors ==
  Bus Element In11 : Inport  PortName=UAVStates  Element=Ve
  Bus Element In12 : Inport  PortName=UAVStates  Element=Xe
  Bus Element In13 : Inport  PortName=UAVStates  Element=pqr
  Bus Element In1 : Inport  PortName=UAVStates  Element=DCMbe
  Bus Element In3 : Inport  PortName=UAVStates  Element=DCMbe
  Bus Element In2 : Inport  PortName=UAVStates  Element=Euler
  Bus Element In4 : Inport  PortName=UAVStates  Element=Abb
  Bus Element In5 : Inport  PortName=UAVStates  Element=airspeed
  Bus Element In6 : Inport  PortName=UAVStates  Element=RotorParameters
  Bus Element In7 : Inport  PortName=UAVStates  Element=Abe
  " Baro Simulation" : Subsystem
  Airspeed : Subsystem
  Bus Creator1 : BusCreator  Inputs=11
  Create States Bus for sensors : Subsystem
  Delay : Delay  DelayLength=1
  GNSS/GPS Simulation : Subsystem
      settings: PortSchema="{\"entries\":[{\"content\":{\"sides\":[{\"content\":{\"connectorIds\":[\"In1\"]},\"type\":\"ConnectorPlacement.EquallySpacedRectSide\",\"uuid\":\"4934e8ff-5d4b-4e11-968d-c23bd62383a0\"},{\"content\":{\"connectorIds\":[\"Out1\",\"Out2\",\"Out3\"],\"side\":\"RIGHT\"},\"type\":\"ConnectorPlacement.EquallySpacedRectSide\",\"uuid\":\"9ec8bc0a-2d3c-4dca-835c-010ac29b6ebc\"},{\"content\":{\"connectorIds\":[],\"side\":\"TOP\"},\"type\":\"ConnectorPlacement.EquallySpacedRectSide\",\"uuid\":\"04f09eb4-1bd9-450e-b951-47054bdd92ad\"},{\"content\":{\"connectorIds\":[\"Out4\"],\"side\":\"BOTTOM\"},\"type\":\"ConnectorPlacement.EquallySpacedRectSide\",\"uuid\":\"54bba437-6d13-4ada-8e8d-b8e04495ee78\"}]},\"type\":\"ConnectorPlacement.EquallySpacedConnector\",\"uuid\":\"9a5920cf-a58d-4c98-839b-fbac94edbe7e\"}],\"packageUris\":[\"http://schema.mathworks.com/mf0/Connector/R2020b\"],\"version\":\"1.0\"}"
  IMU Simulation : Subsystem
  Matrix Multiply : Product  Multiplication=Matrix(*)
  Matrix Multiply1 : Product  Multiplication=Matrix(*)
  Rate Transition : RateTransition  OutPortSampleTime=0.001
  Terminator : Terminator
  Transpose : Math  Operator=transpose
  Transpose1 : Math  Operator=transpose
  ypr : Selector  InputPortWidth=3  IndexOptions=Index vector (dialog)  Indices=[3 2 1]  OutputSizes=1
  SensorData : Outport
  wires:
  GNSS/GPS Simulation/2(GndSpeed) -> Bus Creator1/5  "GPSGroundSpeed"
  Rate Transition/1 -> Delay/1
  Bus Element In1/1 -> Transpose/1
  Bus Element In13/1 -> Matrix Multiply/2
  IMU Simulation/1(Acc) -> Bus Creator1/1  "Abb"
  IMU Simulation/2(Gyro) -> Bus Creator1/2  "Gyro"
  [BarometerPressure] -> Bus Creator1/9  "BarometerPress"
  Bus Element In11/1 -> Create States Bus for sensors/1(Ve)
  GNSS/GPS Simulation/3(Course) -> Bus Creator1/6  "GPSCourse"
  " Baro Simulation"/2(rho) -> Bus Creator1/11, Airspeed/2(rho)  "rho"
  GNSS/GPS Simulation/4(LLA) -> Bus Creator1/8, " Baro Simulation"/1(GPS Position)  "LLA"
  Transpose1/1 -> Matrix Multiply1/1
  Delay/1 -> IMU Simulation/1(States), GNSS/GPS Simulation/1(States), Airspeed/1(States)
  Bus Element In6/1 -> Bus Creator1/10  "RotorParameters"
  [DiffPressure] -> Bus Creator1/7  "DiffPress"
  Bus Element In12/1 -> Create States Bus for sensors/2(Xe)
  Create States Bus for sensors/1(States) -> Rate Transition/1
  " Baro Simulation"/1(Pressure) -> [BarometerPressure]
  Bus Element In5/1 -> Create States Bus for sensors/6(Airspeed)  "airspeed"
  Matrix Multiply/1 -> Create States Bus for sensors/3(pqr_e)
  GNSS/GPS Simulation/1(Velocity) -> Bus Creator1/4  "GPSVelocity"
  Bus Element In2/1 -> ypr/1
  IMU Simulation/3(Mag) -> Bus Creator1/3  "Mag"
  Bus Element In7/1 -> Matrix Multiply1/2
  Airspeed/1(Diff Pressure) -> [DiffPressure]
  Matrix Multiply1/1 -> Create States Bus for sensors/5(acc_lnav_e)
  ypr/1 -> Create States Bus for sensors/4(ypr)
  Bus Element In3/1 -> Transpose1/1
  Transpose/1 -> Matrix Multiply/1
  Bus Element In4/1 -> Terminator/1
  Bus Creator1/1 -> SensorData/1

== system eVTOL_System/Flight Controller/Autopilot/Filter or Estimator ==
  SensorData : Inport
  States : Outport
  wires:
  SensorData/1 -> States/1

== system eVTOL_System/Flight Controller/Autopilot/Fixed Wing Controller ==
  States : Inport
  Control Mode : Inport  Port=2
  AAC SP : Inport  Port=3
  FixedWingSP : Inport  Port=4
  AERT : Inport  Port=5
  Fixed Wing Controller Simulation : Subsystem  VariantControl=TuningMode == 0
  Fixed Wing Controller Tuning : Subsystem  VariantControl=TuningMode ~= 0
  Actuator : Outport

== system eVTOL_System/Flight Controller/Autopilot/Manual Control ==
  Bus Creator : BusCreator  Inputs=4
  Constant{,1..3} (4 alike) : Constant  Value=0
  AERT : Outport
  wires:
  Constant/1 -> Bus Creator/1  "aileron"
  Constant1/1 -> Bus Creator/2  "throttle"
  Constant2/1 -> Bus Creator/3  "elevator"
  Constant3/1 -> Bus Creator/4  "rudder"
  Bus Creator/1 -> AERT/1

== system eVTOL_System/Flight Controller/Autopilot/Multicopter Controller ==
  note: Prefilter
  Hover Commands : Inport
  InTransition : Inport  Port=2
  States : Inport  Port=3
  Altitude Control : Subsystem
  Attitude Control : Subsystem  Variant=on  VariantControlMode=label  VariantControl=Choice  LabelModeActiveChoice=AttitudeControl==1
  Attitude Stabilization : Subsystem  TreatAsAtomicUnit=on
  Demux1 : Demux
  Discrete Transfer Fcn{1..4} (4 alike) : DiscreteTransferFcn  Numerator=ReferenceFilterNum  Denominator=ReferenceFilterDen
  Horizontal Position Control : Subsystem  TreatAsAtomicUnit=on
  Merge : Merge
  Merge1 : Merge
  Mux : Mux  Inputs=3
  NOT1 : Logic  Operator=NOT  IconShape=distinctive  AllPortsSameDT=off  OutDataTypeStr=boolean
  Organize Inputs : Subsystem
  Pitch Ref : Constant  Value=0
  Scope : Scope
  Subsystem : Subsystem
  Variant Source : VariantSource
  Variant Source1 : VariantSource
  MixerCommands : Outport
  wires:
  [Transition] -> NOT1/1
  [State] -> Horizontal Position Control/3(States)
  Variant Source1/1 -> Mux/1
  States/1 -> [State]
  Hover Commands/1 -> Demux1/1
  InTransition/1 -> [Transition]
  NOT1/1 -> Horizontal Position Control/Enable
  [YRef] -> Horizontal Position Control/2(YRef)
  [XRef] -> Horizontal Position Control/1(XRef)
  Attitude Control/1(Roll torque cmd) -> Organize Inputs/2(commanded phi torque)
  [Transition] -> Attitude Stabilization/Enable
  Demux1/3 -> Discrete Transfer Fcn2/1
  Demux1/1 -> Discrete Transfer Fcn3/1
  [State] -> Altitude Control/2(States)
  Demux1/2 -> Discrete Transfer Fcn4/1
  Discrete Transfer Fcn3/1 -> [XRef]
  Demux1/4 -> Discrete Transfer Fcn1/1
  Horizontal Position Control/1(Roll Cmd) -> Variant Source1/1, Merge1/1
  Horizontal Position Control/2(Tilt Cmd) -> Merge/1, Variant Source/1
  Attitude Control/3(Yaw torque Cmd) -> Organize Inputs/4(commanded psi torque)
  Attitude Stabilization/1(Tilt Cmd) -> Merge/2
  Attitude Control/2(Pitch torque Cmd) -> Organize Inputs/3(commanded theta torque)
  Attitude Stabilization/2(Roll Cmd) -> Merge1/2
  Discrete Transfer Fcn4/1 -> [YRef]
  Merge/1 -> Variant Source/2
  Merge1/1 -> Variant Source1/2
  [Transition] -> Subsystem/1(inTransition)
  [State] -> Subsystem/2(States)
  [YawRef] -> Subsystem/3(Reference)
  Variant Source/1 -> Organize Inputs/1(forward command)
  Pitch Ref/1 -> Mux/2
  Subsystem/1(Yaw Reference) -> Mux/3
  Mux/1 -> Attitude Control/1(Ref Attitude)
  [State] -> Attitude Control/2(States)
  [Transition] -> Attitude Control/3(inTransition)
  [ZRef] -> Altitude Control/1(Z ref)
  [Transition] -> Altitude Control/3(InTransition)
  Altitude Control/1(commanded thrust) -> Organize Inputs/5(commanded thrust)
  Organize Inputs/1(MixerCommands) -> MixerCommands/1
  Discrete Transfer Fcn1/1 -> Scope/1, [YawRef]
  Discrete Transfer Fcn2/1 -> [ZRef]

== system eVTOL_System/Flight Controller/Autopilot/Scheduler ==
  MotorCommands : Inport
  TiltSchedule : Inport  Port=2
  FlightState : Inport  Port=3  OutDataTypeStr=Enum: flightState
  States : Inport  Port=4
  TransitionDone : Inport  Port=5
  FixedWingActuators : Inport  Port=6
  Subsystem : Subsystem  ReferencedSubsystem=FixedWingScheduler
  Subsystem1 : Subsystem  ReferencedSubsystem=MulticopterScheduler
  MotorActuatorCommands : Outport
  CtrlSurfaceCommands : Outport  Port=2  VectorParamsAs1DForOutWhenUnconnected=off
  wires:
  Subsystem/1 -> Subsystem1/2, CtrlSurfaceCommands/1
  FlightState/1 -> Subsystem/1, Subsystem1/1  "Flight State"
  TiltSchedule/1 -> Subsystem1/4
  Subsystem1/1 -> MotorActuatorCommands/1
  MotorCommands/1 -> Subsystem1/3
  FixedWingActuators/1 -> Subsystem/2
  TransitionDone/1 -> Subsystem/3, Subsystem1/5  "Transition Done"
  States/1 -> Subsystem1/6

== system eVTOL_System/Flight Controller/Autopilot/Tilt Scheduler ==
  note: Forward Transition Tilt Mode Manager
  note: Back Transition Tilt Mode Manager
  FlightMode : Inport
  States : Inport  Port=2
  Back Transition Scheduler : Subsystem
  Forward Transition Scheduler : Subsystem
  TiltAngle : Outport
  FlightState : Outport  Port=2
  wires:
  States/1 -> Back Transition Scheduler/3(States)
  Back Transition Scheduler/1(TiltAngle) -> TiltAngle/1
  FlightMode/1 -> Back Transition Scheduler/2(FlightMode), Forward Transition Scheduler/1(FlightMode)
  Forward Transition Scheduler/1(FlightState) -> FlightState/1
  Forward Transition Scheduler/2(Tilt Schedule) -> Back Transition Scheduler/1(Tilt Schedule)

== system eVTOL_System/Flight Controller/Estimator/Estimation Filter ==
  Bus Element In : Inport  PortName=SensorData  Element=Abb
  Bus Element In1 : Inport  PortName=SensorData  Element=Gyro
  Bus Element In2 : Inport  PortName=SensorData  Element=Mag
  Bus Element In3 : Inport  PortName=SensorData  Element=GPSVelocity
  Bus Element In4 : Inport  PortName=SensorData  Element=LLA
  Bus Element In6 : Inport  PortName=SensorData  Element=rho
  Bus Element In5 : Inport  PortName=SensorData  Element=DiffPress
  Bus Element In7 : Inport  PortName=SensorData  Element=GPSGroundSpeed
  Bus Element In8 : Inport  PortName=SensorData  Element=GPSCourse
  Bus Element In9 : Inport  PortName=SensorData  Element=RotorParameters
  Bus Element In10 : Inport  PortName=SensorData  Element=BarometerPress
  AHRS1 : mspfiltlib/AHRS  DispRefFrame=NED  DecimationFactor=1  InitialProcessNoise=ahrsfilter.defaultProcessNoise  OrientationFormat=quaternion  SimulateUsing=Code generation  AccelerometerNoise=0.0001924722  GyroscopeNoise=9.1385e-5  MagnetometerNoise=0.1  GyroscopeDriftNoise=3.0462e-13  LinearAccelerationNoise=0.0096236100000000012  MagneticDisturbanceNoise=0.5  LinearAccelerationDecayFactor=0.998  MagneticDisturbanceDecayFactor=0.5  ExpectedMagneticFieldStrength=40
  Airspeed Filter : Subsystem
  Bus Creator : BusCreator  Inputs=13
  Coordinate Transformation Conversion1 : robotcorelib/Coordinate Transformation Conversion  InputRepresentation=Quaternion  InputEulerSequence=ZYX  ShowTrVecInputPort=on  OutputRepresentation=Euler Angles  OutputEulerSequence=ZYX  ShowTrVecOutputPort=on  SimulateUsing=Interpreted execution
      settings: LibrarySourceBlock=navlib/Utilities/Coordinate Transformation Conversion
  Coordinate Transformation Conversion2 : robotcorelib/Coordinate Transformation Conversion  InputRepresentation=Quaternion  InputEulerSequence=ZYX  ShowTrVecInputPort=on  OutputRepresentation=Rotation Matrix  OutputEulerSequence=ZYX  ShowTrVecOutputPort=on  SimulateUsing=Interpreted execution
      settings: LibrarySourceBlock=navlib/Utilities/Coordinate Transformation Conversion
  Degrees to Radians : simulink_extras/Transformations/Degrees to Radians
  Gain : Gain
  LLA2Local : Subsystem
  Matrix Multiply1 : Product  Multiplication=Matrix(*)
  Rate Transition : RateTransition  OutPortSampleTime=0.001
  Rate Transition1 : RateTransition
  Terminator : Terminator
  Transpose{,1..3} (4 alike) : Math  Operator=transpose
  ypr1 : Selector  InputPortWidth=3  IndexOptions=Index vector (dialog)  Indices=[3 2 1]  OutputSizes=1
  EstimatedStates : Outport
  wires:
  AHRS1/2 -> Transpose2/1  "pqr"
  Bus Element In/1 -> AHRS1/1
  Bus Element In1/1 -> AHRS1/2
  Bus Element In2/1 -> AHRS1/3
  Transpose2/1 -> Bus Creator/1  "pqr"
  AHRS1/1 -> Transpose3/1, Transpose1/1, Bus Creator/2  "q"
  Transpose1/1 -> Coordinate Transformation Conversion1/1  "pqr"
  Coordinate Transformation Conversion1/1 -> Bus Creator/3, ypr1/1  "ypr"
  Bus Element In3/1 -> Transpose/1, Bus Creator/8, Gain/1  "Ve_ground"
  Coordinate Transformation Conversion2/1 -> Bus Creator/5, Matrix Multiply1/1  "DCMbe"
  Bus Element In4/1 -> LLA2Local/1(LLA)
  LLA2Local/1(Xe) -> Bus Creator/9  "Xe"
  Matrix Multiply1/1 -> Bus Creator/6  "Vb"
  Bus Element In8/1 -> Degrees to Radians/1
  Bus Element In7/1 -> Bus Creator/11  "gndspeed"
  Bus Element In10/1 -> Terminator/1  "BarometerPress"
  Bus Element In5/1 -> Airspeed Filter/1(DiffPress)
  Bus Element In9/1 -> Rate Transition/1
  Bus Element In6/1 -> Airspeed Filter/2(rho)
  Airspeed Filter/1(airspeed) -> Bus Creator/13  "airspeed"
  ypr1/1 -> Bus Creator/4  "Euler"
  Transpose3/1 -> Coordinate Transformation Conversion2/1  "pqr"
  Degrees to Radians/1 -> Bus Creator/10  "course"
  Rate Transition/1 -> Bus Creator/12  "RotorParameters"
  Transpose/1 -> Matrix Multiply1/2
  Bus Creator/1 -> Rate Transition1/1
  Rate Transition1/1 -> EstimatedStates/1
  Gain/1 -> Bus Creator/7  "Ve"

== system eVTOL_System/Flight Controller/Estimator/Ground Truth ==
  SensorData : Inport
  Rate Transition : RateTransition  OutPortSampleTime=0.005
  EstimatedStates : Outport
  wires:
  SensorData/1 -> Rate Transition/1
  Rate Transition/1 -> EstimatedStates/1

== system eVTOL_System/Flight Controller/Ground Control Station/Get Flight Mission ==
  UAVState : Inport
  noQGC : Subsystem  TreatAsAtomicUnit=on  SystemSampleTime=UAVSampleTime*4  VariantControl=useQGC==0
  "Mission " : Outport

== system eVTOL_System/Flight Controller/Guidance Test Bench/ControlType ==
  Aircraft States : Inport
  Global Mission : Inport  Port=2
  Guidance Testbench : Subsystem  TreatAsAtomicUnit=on  VariantControl=TestMode==1
  Manual Control : Subsystem  TreatAsAtomicUnit=on  VariantControl=TestMode==0
  HoverCmds : Outport
  FixedWingSP : Outport  Port=2
  AACSP : Outport  Port=3
  ctrlMode : Outport  Port=4
  FlightMode : Outport  Port=5

== system eVTOL_System/Flight Controller/Guidance Test Bench/Reference Tracking  ==
  State : Inport
  Position Command : Inport  Port=2
  AAC Commands : Inport  Port=3
  Fixed Wing Reference : Subsystem
  Hover Reference : Subsystem
  Transition Reference : Subsystem
  wires:
  State/1 -> Transition Reference/1(States), Fixed Wing Reference/2(States), Hover Reference/2(Position Reference)
  AAC Commands/1 -> Fixed Wing Reference/1(AAC Commands)
  Position Command/1 -> Hover Reference/1(Position Command)

== system eVTOL_System/Motor Drive/Controller/Controller_HIL_CAN ==
  Iab : Inport
  QAE_MIL_fbk : Inport  Port=2
  EnablePWM : Inport  Port=3
  Closed_Loop_FOC : Inport  Port=4
  Speed_CMD_RPM : Inport  Port=5
  Controller_Parameters : Inport  Port=6
  CAN Communication 611 : Subsystem
  Data Type Conversion : DataTypeConversion  OutDataTypeStr=uint8  SaturateOnIntegerOverflow=off  RndMeth=Floor
  Data Type Conversion1 : DataTypeConversion  OutDataTypeStr=uint8  SaturateOnIntegerOverflow=off  RndMeth=Floor
  Data Type Conversion2 : DataTypeConversion  OutDataTypeStr=single  SaturateOnIntegerOverflow=off  RndMeth=Floor
  Internal PWM configuration1 : Subsystem
  Mux : Mux
  Terminator8 : Terminator
  Terminator9 : Terminator
  Simu_config : Outport
  Controller_fbk : Outport  Port=2
  wires:
  Iab/1 -> Terminator9/1
  Speed_CMD_RPM/1 -> CAN Communication 611/1(Speed_CMD_rpm)
  Controller_Parameters/1 -> CAN Communication 611/4(Controller_Parameters)
  EnablePWM/1 -> Data Type Conversion1/1
  Data Type Conversion/1 -> CAN Communication 611/2(Closed_loop)
  QAE_MIL_fbk/1 -> Terminator8/1
  Closed_Loop_FOC/1 -> Data Type Conversion/1
  Data Type Conversion1/1 -> CAN Communication 611/3(EnablePWM)
  Data Type Conversion2/1 -> Controller_fbk/1
  CAN Communication 611/2(Pos_fdk) -> Mux/2
  CAN Communication 611/1(Speed_fbk) -> Mux/1
  CAN Communication 611/4(Spd_pot) -> Mux/4
  CAN Communication 611/3(Speed_Cmd) -> Mux/3
  Mux/1 -> Data Type Conversion2/1
  Internal PWM configuration1/1(Simu Config) -> Simu_config/1

== system eVTOL_System/Motor Drive/Controller/Controller_MIL ==
  Iab : Inport
  QAE_MIL_fbk : Inport  Port=2
  EnablePWM : Inport  Port=3
  Closed_Loop_FOC : Inport  Port=4
  Speed_CMD_RPM : Inport  Port=5
  Controller_Parameters : Inport  Port=6
  Bus Creator : BusCreator  Inputs=5
  Bus Selector : BusSelector  OutputSignals=Ia_offset,Ib_offset,Kp_S,Ki_S,Kp_I,Ki_IxTcpu
  Constant : Constant  Value=0  OutDataTypeStr=single  SampleTime=Ts_CPU
  Constant4 : Constant
  Data Type Conversion : DataTypeConversion  SaturateOnIntegerOverflow=off  RndMeth=Floor
  Data Type Conversion1 : DataTypeConversion  OutDataTypeStr=double  SaturateOnIntegerOverflow=off  RndMeth=Floor
  Data Type Conversion2 : DataTypeConversion  OutDataTypeStr=boolean  SaturateOnIntegerOverflow=off  RndMeth=Floor
  Data Type Conversion3 : DataTypeConversion  SaturateOnIntegerOverflow=off  RndMeth=Floor
  Data Type Conversion4 : DataTypeConversion  OutDataTypeStr=boolean  SaturateOnIntegerOverflow=off  RndMeth=Floor
  Data Type Conversion6 : DataTypeConversion  OutDataTypeStr=uint16  RndMeth=Simplest  SaturateOnIntegerOverflow=off
  F28379D ADC : Subsystem
  F28379D Firmware : Subsystem
  IO334 DAC : Subsystem
  Mux : Mux  Inputs=3
  PWM Generation : pwm_cpulib/PWM Generation  f_FPGA=f_FPGA  n_channels=3  sel_scaling=CPU  protection_param=A/B are forced off when A/B are on.  deadband_sec=0  natural_update=At period starts  delay=0  trigger_duration_sec=[1e-6]  trigger_period_start=off  trigger_half_of_the_period=off  trigger_a_on=off  trigger_a_off=off  trigger_b_on=off  trigger_b_off=off  bit_width_pwm_gen=24  invert_a=off  invert_b=off  invert_c=off  showPhaseInput=off
      settings: SourceProductName=PWM CPU Library
  PWM Periods : Constant  Value=[1/PWM_frequency 1/PWM_frequency 1/PWM_frequency]  OutDataTypeStr=double  SampleTime=-1
  Rate Transition1 : RateTransition  OutPortSampleTime=Ts_speed
  Rate Transition12 : RateTransition  OutPortSampleTime=Ts_UI
  Rate Transition{2,4..9} (7 alike) : RateTransition  OutPortSampleTime=Ts_CPU
  Rate Transition3 : RateTransition  OutPortSampleTime=Ts_speed
  bias1 : Constant  OutDataTypeStr=boolean  SampleTime=Ts_CPU
  bias3 : Constant  Value=0  OutDataTypeStr=boolean  SampleTime=Ts_CPU
  Simu_config : Outport
  Controller_fbk : Outport  Port=2
  wires:
  bias1/1 -> Bus Creator/1  "PCIe_RC_or_TTL"
  Bus Creator/1 -> Simu_config/1
  Constant4/1 -> Data Type Conversion6/1
  Data Type Conversion/1 -> Bus Creator/4  "PCIe_PWM_Enable"
  Iab/1 -> IO334 DAC/1(Iab)
  IO334 DAC/1(Iab_IO334DAC) -> F28379D ADC/1(Iab_IO334V)  "IabV"
  F28379D ADC/1(Ia_ADC) -> F28379D Firmware/1(Ia_ADC)
  F28379D ADC/2(Ib_ADC) -> F28379D Firmware/2(Ib_ADC)
  QAE_MIL_fbk/1 -> F28379D Firmware/5(QEP_Position_Count)
  Data Type Conversion6/1 -> F28379D Firmware/6(QEP_Index_Latch)
  Bus Selector/3 -> Rate Transition3/1  "<Kp_S>"
  F28379D Firmware/2(PWM_Enable) -> Data Type Conversion/1
  Data Type Conversion2/1 -> F28379D Firmware/11(EnablePWM)
  Data Type Conversion4/1 -> F28379D Firmware/10(EnClosedLoop)
  Bus Selector/4 -> Rate Transition1/1  "<Ki_S>"
  Closed_Loop_FOC/1 -> Rate Transition4/1
  Controller_Parameters/1 -> Bus Selector/1
  Bus Selector/1 -> Rate Transition5/1  "<Ia_offset>"
  Bus Selector/2 -> Rate Transition6/1  "<Ib_offset>"
  Bus Selector/5 -> Rate Transition8/1  "<Kp_I>"
  Bus Selector/6 -> Rate Transition9/1  "<Ki_IxTcpu>"
  EnablePWM/1 -> Rate Transition7/1
  Mux/1 -> Rate Transition12/1
  F28379D Firmware/3(Fbk_CAN) -> Mux/1
  Speed_CMD_RPM/1 -> Rate Transition2/1
  Rate Transition3/1 -> F28379D Firmware/8(Kp_S)
  Rate Transition1/1 -> F28379D Firmware/9(Ki_S)
  Rate Transition5/1 -> F28379D Firmware/3(IaOffset)
  Rate Transition6/1 -> F28379D Firmware/4(IbOffset)
  Rate Transition4/1 -> Data Type Conversion4/1
  Rate Transition7/1 -> Data Type Conversion2/1
  Rate Transition8/1 -> F28379D Firmware/12(Kp_i)
  Rate Transition9/1 -> F28379D Firmware/13(Ki_ixTcpu)
  Rate Transition12/1 -> Controller_fbk/1
  Constant/1 -> Mux/3
  Rate Transition2/1 -> F28379D Firmware/7(SpdCmdRPM), Mux/2
  bias3/1 -> Bus Creator/5  "PCIe_Protocol"
  PWM Periods/1 -> PWM Generation/1
  PWM Generation/1 -> Bus Creator/2  "PCIe_PWM_Config"
  PWM Generation/2 -> Data Type Conversion3/1  "PCIe_PWM_Runtime"
  Data Type Conversion1/1 -> PWM Generation/2
  F28379D Firmware/1(ModWave) -> Data Type Conversion1/1
  Data Type Conversion3/1 -> Bus Creator/3  "PCIe_PWM_Runtime"
